simulink model "supply_fan_speed_logic"  (R2020b)
settings: Solver=VariableStepAuto  StartTime=0.0  StopTime=10.0  RelTol=1e-3
undefined symbols (not defined in the file): fan_speed_enum
libraries: simulink x1
settings Model: DataDictionary=airsys_data_dict.sldd  Creator=Litao  LastModifiedBy=Litao

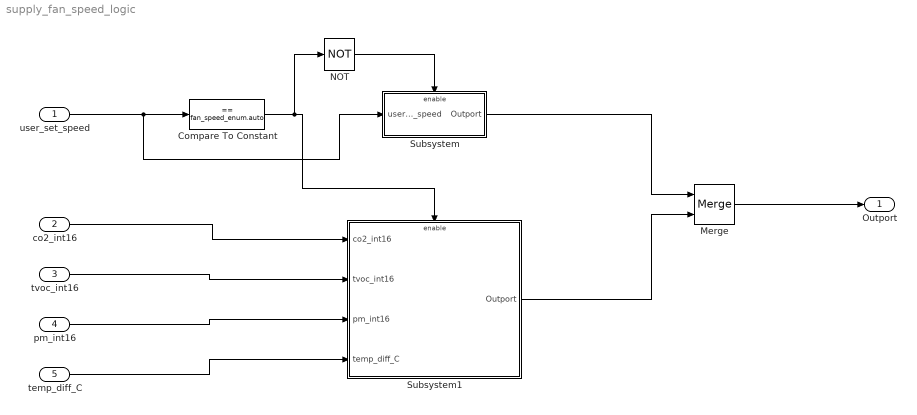
== system supply_fan_speed_logic ==
  user_set_speed : Inport  OutDataTypeStr=Enum: fan_speed_enum
  co2_int16 : Inport  Port=2  OutDataTypeStr=uint16
  tvoc_int16 : Inport  Port=3  OutDataTypeStr=uint16
  pm_int16 : Inport  Port=4  OutDataTypeStr=uint16
  temp_diff_C : Inport  Port=5  OutDataTypeStr=double
  Compare To Constant : simulink/Logic and Bit Operations/Compare To Constant  relop===  const=fan_speed_enum.auto  OutDataTypeStr=boolean
  Merge : Merge
  NOT : Logic  Operator=NOT  IconShape=distinctive  AllPortsSameDT=off  OutDataTypeStr=boolean
  Subsystem : Subsystem
  Subsystem1 : Subsystem
  Outport : Outport
  wires:
  user_set_speed/1 -> Subsystem/1(user_set_speed), Compare To Constant/1
  NOT/1 -> Subsystem/Enable
  Compare To Constant/1 -> Subsystem1/Enable, NOT/1
  co2_int16/1 -> Subsystem1/1(co2_int16)
  tvoc_int16/1 -> Subsystem1/2(tvoc_int16)
  pm_int16/1 -> Subsystem1/3(pm_int16)
  temp_diff_C/1 -> Subsystem1/4(temp_diff_C)
  Merge/1 -> Outport/1
  Subsystem/1(Outport) -> Merge/1
  Subsystem1/1(Outport) -> Merge/2

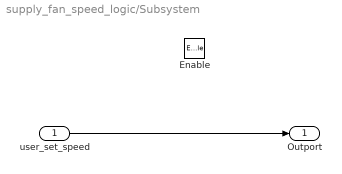
== system supply_fan_speed_logic/Subsystem ==
  user_set_speed : Inport
  Enable : EnablePort
  Outport : Outport
  wires:
  user_set_speed/1 -> Outport/1

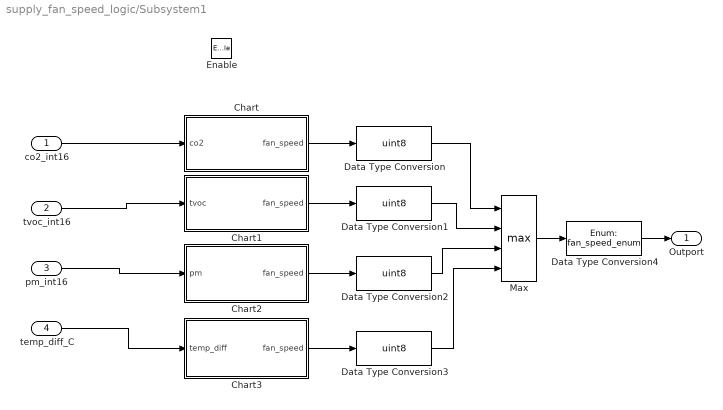
== system supply_fan_speed_logic/Subsystem1 ==
  co2_int16 : Inport
  tvoc_int16 : Inport  Port=2
  pm_int16 : Inport  Port=3
  temp_diff_C : Inport  Port=4
  Enable : EnablePort
  Chart : Stateflow chart  TreatAsAtomicUnit=on
  Chart1 : Stateflow chart  TreatAsAtomicUnit=on
  Chart2 : Stateflow chart  TreatAsAtomicUnit=on
  Chart3 : Stateflow chart  TreatAsAtomicUnit=on
  Data Type Conversion{,1..3} (4 alike) : DataTypeConversion  OutDataTypeStr=uint8
  Data Type Conversion4 : DataTypeConversion  OutDataTypeStr=Enum: fan_speed_enum
  Max : MinMax  Function=max  Inputs=4
  Outport : Outport
  wires:
  co2_int16/1 -> Chart/1(co2)
  tvoc_int16/1 -> Chart1/1(tvoc)
  pm_int16/1 -> Chart2/1(pm)
  temp_diff_C/1 -> Chart3/1(temp_diff)
  Chart/1(fan_speed) -> Data Type Conversion/1
  Chart1/1(fan_speed) -> Data Type Conversion1/1
  Chart2/1(fan_speed) -> Data Type Conversion2/1
  Chart3/1(fan_speed) -> Data Type Conversion3/1
  Max/1 -> Data Type Conversion4/1
  Data Type Conversion/1 -> Max/1
  Data Type Conversion1/1 -> Max/2
  Data Type Conversion2/1 -> Max/3
  Data Type Conversion3/1 -> Max/4
  Data Type Conversion4/1 -> Outport/1

== stateflow chart supply_fan_speed_logic/Subsystem1/Chart1 ==
  state high
    du:fan_speed=fan_speed_enum.high
  state mid
    du:fan_speed=fan_speed_enum.mid
  state low
    du:fan_speed=fan_speed_enum.low
  mid -> high [order 2] : [tvoc>2000]
  high -> mid : [tvoc<1900]
  low -> mid : [tvoc>1000]
  mid -> low [order 1] : [tvoc<900]
  (default) -> low
  data: tvoc input; fan_speed output

== stateflow chart supply_fan_speed_logic/Subsystem1/Chart2 ==
  state high
    du:fan_speed=fan_speed_enum.high
  state mid
    du:fan_speed=fan_speed_enum.mid
  state low
    du:fan_speed=fan_speed_enum.low
  mid -> high [order 2] : [pm>125]
  high -> mid : [pm<100]
  low -> mid : [pm>75]
  mid -> low [order 1] : [pm<50]
  (default) -> low
  data: fan_speed output; pm input

== stateflow chart supply_fan_speed_logic/Subsystem1/Chart ==
  state high
    du:fan_speed=fan_speed_enum.high
  state mid
    du:fan_speed=fan_speed_enum.mid
  state low
    du:fan_speed=fan_speed_enum.low
  mid -> high [order 2] : [co2>2000]
  high -> mid : [co2<1900]
  low -> mid : [co2>1000]
  mid -> low [order 1] : [co2<900]
  (default) -> low
  data: co2 input; fan_speed output

== stateflow chart supply_fan_speed_logic/Subsystem1/Chart3 ==
  state high
    du:fan_speed=fan_speed_enum.high
  state mid
    du:fan_speed=fan_speed_enum.mid
  state low
    du:fan_speed=fan_speed_enum.low
  mid -> high [order 2] : [temp_diff>4]
  high -> mid : [temp_diff<3]
  low -> mid : [temp_diff>2]
  mid -> low [order 1] : [temp_diff<1]
  (default) -> low
  data: fan_speed output; temp_diff input
